simulink model "Plugin_NLPID"  (Simulink 7.3)
settings: Solver=ode45  StartTime=0.0  StopTime=10.0  RelTol=1e-3
libraries: dspmtrx3 x5
settings Model: Creator=mcl  LastModifiedBy=mcl

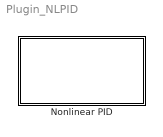
== system Plugin_NLPID ==
  Nonlinear PID : Subsystem

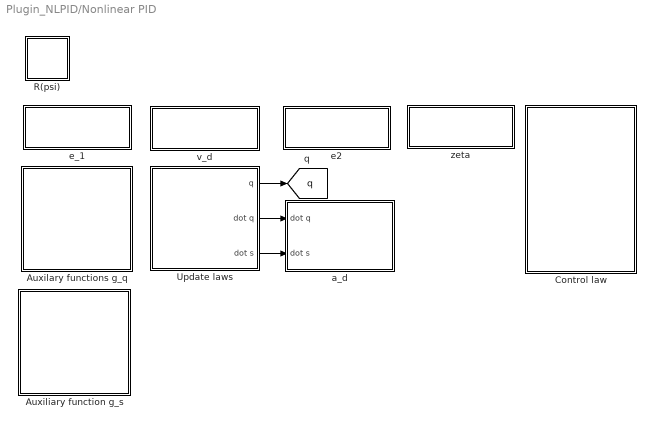
== system Plugin_NLPID/Nonlinear PID ==
  Auxilary functions g_q : Subsystem
  Auxiliary function g_s : Subsystem
  Control law : Subsystem
  R(psi) : Subsystem
  Update laws : Subsystem
  a_d : Subsystem
  e2 : Subsystem
  e_1 : Subsystem
  v_d : Subsystem
  zeta : Subsystem
  tag scope: q=global
  wires:
  Update laws/1(q) -> [q]
  Update laws/2(dot q) -> a_d/1(dot q)
  Update laws/3(dot s) -> a_d/2(dot s)

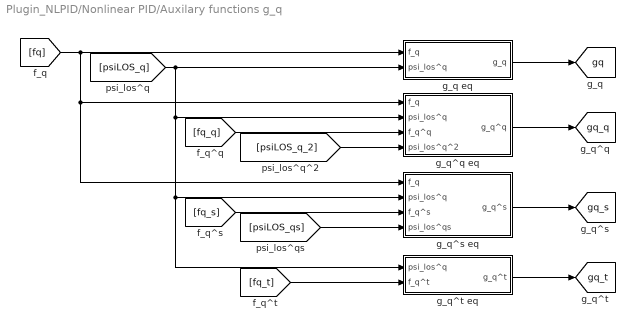
== system Plugin_NLPID/Nonlinear PID/Auxilary functions g_q ==
  g_q eq : Subsystem
  g_q^q eq : Subsystem
  g_q^s eq : Subsystem
  g_q^t eq : Subsystem
  tag scope: gq=global, gq_q=global, gq_s=global, gq_t=global
  wires:
  [fq_t] -> g_q^t eq/2(f_q^t)
  g_q^t eq/1(g_q^t) -> [gq_t]
  [psiLOS_qs] -> g_q^s eq/4(psi_los^qs)
  [fq_s] -> g_q^s eq/3(f_q^s)
  g_q^s eq/1(g_q^s) -> [gq_s]
  g_q^q eq/1(g_q^q) -> [gq_q]
  [psiLOS_q_2] -> g_q^q eq/4(psi_los^q^2)
  [fq_q] -> g_q^q eq/3(f_q^q)
  [fq] -> g_q^s eq/1(f_q), g_q^q eq/1(f_q), g_q eq/1(f_q)
  [psiLOS_q] -> g_q^t eq/1(psi_los^q), g_q^s eq/2(psi_los^q), g_q^q eq/2(psi_los^q), g_q eq/2(psi_los^q)
  g_q eq/1(g_q) -> [gq]

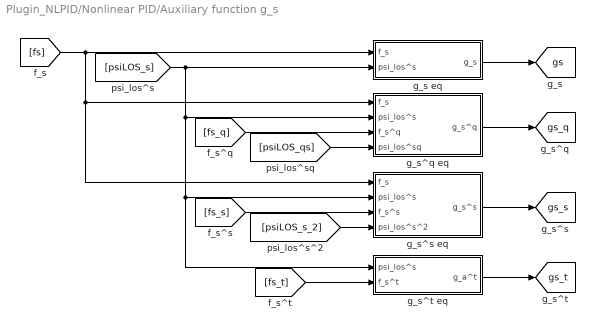
== system Plugin_NLPID/Nonlinear PID/Auxiliary function g_s ==
  g_s eq : Subsystem
  g_s^q eq : Subsystem
  g_s^s eq : Subsystem
  g_s^t eq : Subsystem
  tag scope: gs=global, gs_q=global, gs_s=global, gs_t=global
  wires:
  [fs_t] -> g_s^t eq/2(f_s^t)
  g_s^t eq/1(g_a^t) -> [gs_t]
  [psiLOS_s_2] -> g_s^s eq/4(psi_los^s^2)
  [fs_s] -> g_s^s eq/3(f_s^s)
  g_s^s eq/1(g_s^s) -> [gs_s]
  g_s^q eq/1(g_s^q) -> [gs_q]
  [psiLOS_qs] -> g_s^q eq/4(psi_los^sq)
  [fs_q] -> g_s^q eq/3(f_s^q)
  g_s eq/1(g_s) -> [gs]
  [psiLOS_s] -> g_s^t eq/1(psi_los^s), g_s^s eq/2(psi_los^s), g_s^q eq/2(psi_los^s), g_s eq/2(psi_los^s)
  [fs] -> g_s^s eq/1(f_s), g_s^q eq/1(f_s), g_s eq/1(f_s)

== system Plugin_NLPID/Nonlinear PID/Control law ==
  Product : Product  OutDataType=fixdt(1, 16)  OutScaling=2^0  RndMeth=Zero
  Product1 : Product  OutDataType=fixdt(1, 16)  OutScaling=2^0  RndMeth=Zero
  Sum : Sum  Inputs=+++  OutDataType=fixdt(1, 16)  OutScaling=2^-10
  tau_FF : Subsystem
  tau_FL : Subsystem
  tau_PID : Subsystem
  tag scope: ctrl2tau=global
  wires:
  Sum/1 -> [ctrl2tau]
  tau_PID/1(tau_PID) -> Sum/1
  [tauxscale] -> Product/1
  [tauyscale] -> Product1/1
  tau_FL/1(tau_FL) -> Product/2
  Product/1 -> Sum/2
  tau_FF/1(tau_FF) -> Product1/2
  Product1/1 -> Sum/3

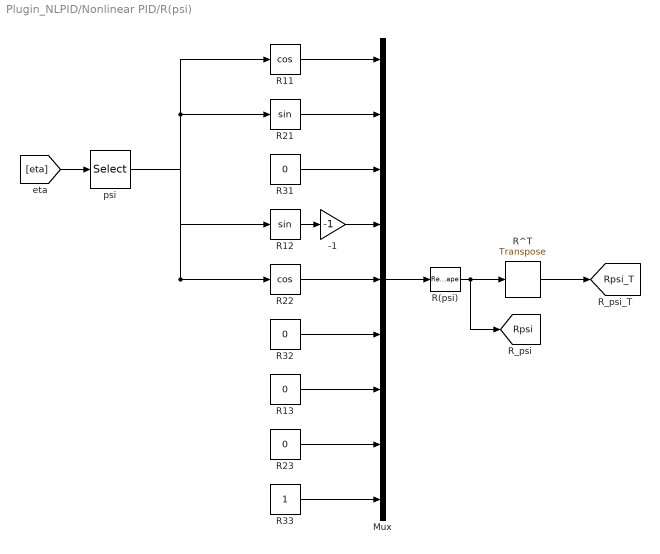
== system Plugin_NLPID/Nonlinear PID/R(psi) ==
  -1 : Gain  Gain=-1  ParameterDataType=fixdt(1, 16)  ParameterScaling=2^0  OutDataType=fixdt(1, 16)  OutScaling=2^0
  Mux : Mux  Inputs=9
  R(psi) : Reshape  OutputDimensionality=Customize  OutputDimensions=[3,3]
  R11 : Trigonometry  Operator=cos
  R12 : Trigonometry
  R{13,23,31..32} (4 alike) : Constant  Value=0
  R21 : Trigonometry
  R22 : Trigonometry  Operator=cos
  R33 : Constant
  R^T : dspmtrx3/Transpose  SystemSampleTime=-1  Hermitian=off  overflowFlag=off
  psi : Selector  InputPortWidth=3  IndexOptions=Index vector (dialog)  Indices=[3]  OutputSizes=1
  tag scope: Rpsi=global, Rpsi_T=global
  wires:
  R(psi)/1 -> [Rpsi], R^T/1
  Mux/1 -> R(psi)/1
  psi/1 -> R11/1, R21/1, R12/1, R22/1
  R11/1 -> Mux/1
  R21/1 -> Mux/2
  R31/1 -> Mux/3
  R12/1 -> -1/1
  R22/1 -> Mux/5
  R32/1 -> Mux/6
  R13/1 -> Mux/7
  R33/1 -> Mux/9
  R23/1 -> Mux/8
  -1/1 -> Mux/4
  [eta] -> psi/1
  R^T/1 -> [Rpsi_T]

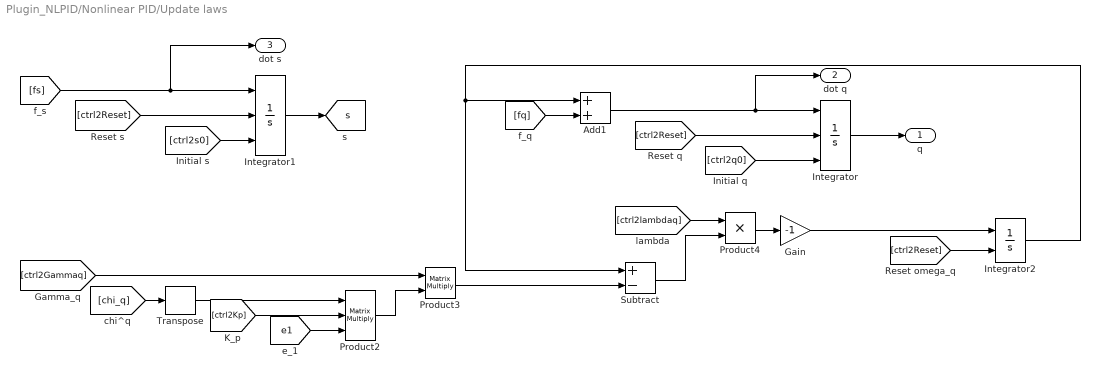
== system Plugin_NLPID/Nonlinear PID/Update laws ==
  Add1 : Sum  OutDataType=fixdt(1, 16)  OutScaling=2^-10
  Gain : Gain  Gain=-1  ParameterDataType=fixdt(1, 16)  ParameterScaling=2^0  OutDataType=fixdt(1, 16)  OutScaling=2^0
  Integrator : Integrator  ExternalReset=level  InitialConditionSource=external
  Integrator1 : Integrator  ExternalReset=level  InitialConditionSource=external  InitialCondition=250
  Integrator2 : Integrator  ExternalReset=level
  Product2 : Product  Inputs=3  Multiplication=Matrix(*)  OutDataType=fixdt(1, 16)  OutScaling=2^0  RndMeth=Zero
  Product3 : Product  Multiplication=Matrix(*)  OutDataType=fixdt(1, 16)  OutScaling=2^0  RndMeth=Zero
  Product4 : Product  OutDataType=fixdt(1, 16)  OutScaling=2^0  RndMeth=Zero
  Subtract : Sum  Inputs=+-  OutDataType=fixdt(1, 16)  OutScaling=2^-10
  Transpose : dspmtrx3/Transpose  SystemSampleTime=-1  Hermitian=off  overflowFlag=off
  q : Outport  PortDimensions=2
  dot q : Outport  Port=2  PortDimensions=2
  dot s : Outport  Port=3  PortDimensions=1
  tag scope: s=global
  wires:
  [chi_q] -> Transpose/1
  [e1] -> Product2/3
  Transpose/1 -> Product2/1
  [ctrl2Kp] -> Product2/2
  [ctrl2Gammaq] -> Product3/1
  Product3/1 -> Subtract/2
  Product2/1 -> Product3/2
  [fs] -> Integrator1/1, dot s/1
  Integrator1/1 -> [s]
  [ctrl2Reset] -> Integrator1/2
  [ctrl2s0] -> Integrator1/3
  [fq] -> Add1/2
  Add1/1 -> Integrator/1, dot q/1
  [ctrl2lambdaq] -> Product4/1
  Subtract/1 -> Product4/2
  Product4/1 -> Gain/1
  Gain/1 -> Integrator2/1
  Integrator/1 -> q/1
  Integrator2/1 -> Add1/1, Subtract/1
  [ctrl2Reset] -> Integrator/2
  [ctrl2q0] -> Integrator/3
  [ctrl2Reset] -> Integrator2/2

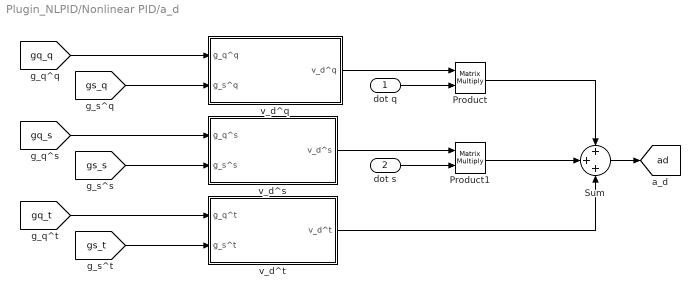
== system Plugin_NLPID/Nonlinear PID/a_d ==
  dot q : Inport
  dot s : Inport  Port=2
  Product : Product  Multiplication=Matrix(*)  OutDataType=fixdt(1, 16)  OutScaling=2^0  RndMeth=Zero
  Product1 : Product  Multiplication=Matrix(*)  OutDataType=fixdt(1, 16)  OutScaling=2^0  RndMeth=Zero
  Sum : Sum  Inputs=+++  OutDataType=fixdt(1, 16)  OutScaling=2^-10
  v_d^q : Subsystem
  v_d^s : Subsystem
  v_d^t : Subsystem
  tag scope: ad=global
  wires:
  v_d^q/1(v_d^q) -> Product/1
  dot q/1 -> Product/2
  Product/1 -> Sum/1
  v_d^s/1(v_d^s) -> Product1/1
  dot s/1 -> Product1/2
  Product1/1 -> Sum/2
  v_d^t/1(v_d^t) -> Sum/3
  Sum/1 -> [ad]
  [gq_q] -> v_d^q/1(g_q^q)
  [gs_q] -> v_d^q/2(g_s^q)
  [gq_s] -> v_d^s/1(g_q^s)
  [gs_s] -> v_d^s/2(g_s^s)
  [gq_t] -> v_d^t/1(g_q^t)
  [gs_t] -> v_d^t/2(g_s^t)

== system Plugin_NLPID/Nonlinear PID/e2 ==
  Product : Product  Multiplication=Matrix(*)  OutDataType=fixdt(1, 16)  OutScaling=2^0  RndMeth=Zero
  Subtract : Sum  Inputs=+-  OutDataType=fixdt(1, 16)  OutScaling=2^-10
  tag scope: e2=global
  wires:
  [nu] -> Subtract/1
  Product/1 -> Subtract/2
  [Rpsi_T] -> Product/1
  [vd] -> Product/2
  Subtract/1 -> [e2]

== system Plugin_NLPID/Nonlinear PID/e_1 ==
  Heading to -pi/pi : Subsystem
  Heading to -pi/pi1 : Subsystem
  Subtract : Sum  Inputs=+-  OutDataType=fixdt(1, 16)  OutScaling=2^-10
  tag scope: e1=global
  wires:
  Subtract/1 -> Heading to -pi/pi1/1(eta rad)
  [eta] -> Heading to -pi/pi/1(eta rad)
  Heading to -pi/pi/1(eta -pi/pi) -> Subtract/1
  Heading to -pi/pi1/1(eta -pi/pi) -> [e1]
  [chi] -> Subtract/2

== system Plugin_NLPID/Nonlinear PID/v_d ==
  Add : Sum  OutDataType=fixdt(1, 16)  OutScaling=2^-10
  tag scope: vd=global
  wires:
  [gq] -> Add/1
  [gs] -> Add/2
  Add/1 -> [vd]

== system Plugin_NLPID/Nonlinear PID/zeta ==
  Integrator : Integrator  ExternalReset=level  InitialCondition=[0 0 0]'
  Product : Product  Multiplication=Matrix(*)  OutDataType=fixdt(1, 16)  OutScaling=2^0  RndMeth=Zero
  tag scope: zeta=global
  wires:
  [ctrl2Reset] -> Integrator/2
  Product/1 -> Integrator/1
  Integrator/1 -> [zeta]
  [e2] -> Product/2
  [Rpsi] -> Product/1

== system Plugin_NLPID/Nonlinear PID/Auxilary functions g_q/g_q eq ==
  f_q : Inport
  psi_los^q : Inport  Port=2
  Product : Product  Multiplication=Matrix(*)  OutDataType=fixdt(1, 16)  OutScaling=2^0  RndMeth=Zero
  Vector Concatenate : Concatenate  Mode=Vector
  g_q : Outport
  wires:
  Product/1 -> Vector Concatenate/2
  psi_los^q/1 -> Product/1
  f_q/1 -> Product/2, Vector Concatenate/1
  Vector Concatenate/1 -> g_q/1

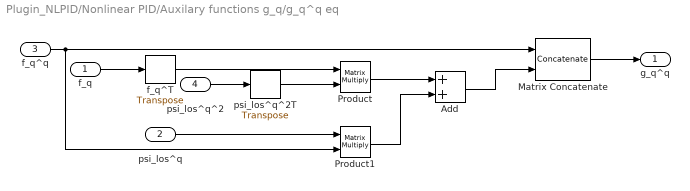
== system Plugin_NLPID/Nonlinear PID/Auxilary functions g_q/g_q^q eq ==
  f_q : Inport
  psi_los^q : Inport  Port=2
  f_q^q : Inport  Port=3
  psi_los^q^2 : Inport  Port=4
  Add : Sum  OutDataType=fixdt(1, 16)  OutScaling=2^-10
  Matrix Concatenate : Concatenate  Mode=Multidimensional array
  Product : Product  Multiplication=Matrix(*)  OutDataType=fixdt(1, 16)  OutScaling=2^0  RndMeth=Zero
  Product1 : Product  Multiplication=Matrix(*)  OutDataType=fixdt(1, 16)  OutScaling=2^0  RndMeth=Zero
  f_q^T : dspmtrx3/Transpose  SystemSampleTime=-1  Hermitian=off  overflowFlag=off
  psi_los^q^2T : dspmtrx3/Transpose  SystemSampleTime=-1  Hermitian=off  overflowFlag=off
  g_q^q : Outport
  wires:
  psi_los^q^2T/1 -> Product/2
  Product1/1 -> Add/2
  psi_los^q/1 -> Product1/1
  Product/1 -> Add/1
  psi_los^q^2/1 -> psi_los^q^2T/1
  f_q^T/1 -> Product/1
  f_q/1 -> f_q^T/1
  Add/1 -> Matrix Concatenate/2
  Matrix Concatenate/1 -> g_q^q/1
  f_q^q/1 -> Product1/2, Matrix Concatenate/1

== system Plugin_NLPID/Nonlinear PID/Auxilary functions g_q/g_q^s eq ==
  f_q : Inport
  psi_los^q : Inport  Port=2
  f_q^s : Inport  Port=3
  psi_los^qs : Inport  Port=4
  Add : Sum  OutDataType=fixdt(1, 16)  OutScaling=2^-10
  Product : Product  Multiplication=Matrix(*)  OutDataType=fixdt(1, 16)  OutScaling=2^0  RndMeth=Zero
  Product1 : Product  Multiplication=Matrix(*)  OutDataType=fixdt(1, 16)  OutScaling=2^0  RndMeth=Zero
  Vector Concatenate : Concatenate  Mode=Vector
  g_q^s : Outport
  wires:
  f_q/1 -> Product/2
  psi_los^qs/1 -> Product/1
  Product1/1 -> Add/2
  psi_los^q/1 -> Product1/1
  Product/1 -> Add/1
  Add/1 -> Vector Concatenate/2
  Vector Concatenate/1 -> g_q^s/1
  f_q^s/1 -> Product1/2, Vector Concatenate/1

== system Plugin_NLPID/Nonlinear PID/Auxilary functions g_q/g_q^t eq ==
  psi_los^q : Inport
  f_q^t : Inport  Port=2
  Product1 : Product  Multiplication=Matrix(*)  OutDataType=fixdt(1, 16)  OutScaling=2^0  RndMeth=Zero
  Vector Concatenate : Concatenate  Mode=Vector
  g_q^t : Outport
  wires:
  psi_los^q/1 -> Product1/1
  Product1/1 -> Vector Concatenate/2
  Vector Concatenate/1 -> g_q^t/1
  f_q^t/1 -> Product1/2, Vector Concatenate/1

== system Plugin_NLPID/Nonlinear PID/Auxiliary function g_s/g_s eq ==
  f_s : Inport
  psi_los^s : Inport  Port=2
  0_2x1 : Constant  Value=[0;0]  VectorParams1D=off  OutDataType=fixdt(1, 16)  OutScaling=2^0
  Product : Product  Multiplication=Matrix(*)  OutDataType=fixdt(1, 16)  OutScaling=2^0  RndMeth=Zero
  Vector Concatenate : Concatenate  Mode=Vector
  g_s : Outport
  wires:
  0_2x1/1 -> Vector Concatenate/1
  Product/1 -> Vector Concatenate/2
  psi_los^s/1 -> Product/1
  f_s/1 -> Product/2
  Vector Concatenate/1 -> g_s/1

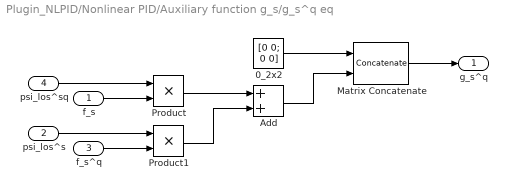
== system Plugin_NLPID/Nonlinear PID/Auxiliary function g_s/g_s^q eq ==
  f_s : Inport
  psi_los^s : Inport  Port=2
  f_s^q : Inport  Port=3
  psi_los^sq : Inport  Port=4
  0_2x2 : Constant  Value=[0 0; 0 0]  VectorParams1D=off  OutDataType=fixdt(1, 16)  OutScaling=2^0
  Add : Sum  OutDataType=fixdt(1, 16)  OutScaling=2^-10
  Matrix Concatenate : Concatenate  Mode=Multidimensional array
  Product : Product  OutDataType=fixdt(1, 16)  OutScaling=2^0  RndMeth=Zero
  Product1 : Product  OutDataType=fixdt(1, 16)  OutScaling=2^0  RndMeth=Zero
  g_s^q : Outport
  wires:
  f_s/1 -> Product/2
  psi_los^sq/1 -> Product/1
  f_s^q/1 -> Product1/2
  0_2x2/1 -> Matrix Concatenate/1
  Product1/1 -> Add/2
  psi_los^s/1 -> Product1/1
  Product/1 -> Add/1
  Add/1 -> Matrix Concatenate/2
  Matrix Concatenate/1 -> g_s^q/1

== system Plugin_NLPID/Nonlinear PID/Auxiliary function g_s/g_s^s eq ==
  f_s : Inport
  psi_los^s : Inport  Port=2
  f_s^s : Inport  Port=3
  psi_los^s^2 : Inport  Port=4
  0_2x1 : Constant  Value=[0;0]  VectorParams1D=off  OutDataType=fixdt(1, 16)  OutScaling=2^0
  Add : Sum  OutDataType=fixdt(1, 16)  OutScaling=2^-10
  Product : Product  OutDataType=fixdt(1, 16)  OutScaling=2^0  RndMeth=Zero
  Product1 : Product  OutDataType=fixdt(1, 16)  OutScaling=2^0  RndMeth=Zero
  Vector Concatenate : Concatenate  Mode=Vector
  g_s^s : Outport
  wires:
  f_s^s/1 -> Product1/2
  0_2x1/1 -> Vector Concatenate/1
  f_s/1 -> Product/2
  psi_los^s^2/1 -> Product/1
  Product1/1 -> Add/2
  psi_los^s/1 -> Product1/1
  Product/1 -> Add/1
  Add/1 -> Vector Concatenate/2
  Vector Concatenate/1 -> g_s^s/1

== system Plugin_NLPID/Nonlinear PID/Auxiliary function g_s/g_s^t eq ==
  psi_los^s : Inport
  f_s^t : Inport  Port=2
  0_2x1 : Constant  Value=[0;0]  VectorParams1D=off  OutDataType=fixdt(1, 16)  OutScaling=2^0
  Product1 : Product  Multiplication=Matrix(*)  OutDataType=fixdt(1, 16)  OutScaling=2^0  RndMeth=Zero
  Vector Concatenate : Concatenate  Mode=Vector
  g_a^t : Outport
  wires:
  f_s^t/1 -> Product1/2
  0_2x1/1 -> Vector Concatenate/1
  psi_los^s/1 -> Product1/1
  Product1/1 -> Vector Concatenate/2
  Vector Concatenate/1 -> g_a^t/1

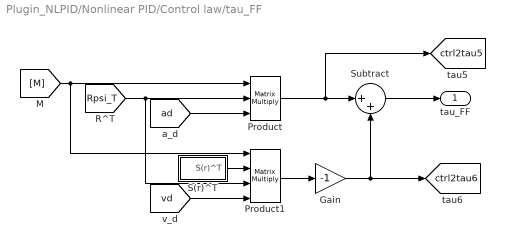
== system Plugin_NLPID/Nonlinear PID/Control law/tau_FF ==
  Gain : Gain  Gain=-1  ParameterDataType=fixdt(1, 16)  ParameterScaling=2^0  OutDataType=fixdt(1, 16)  OutScaling=2^0
  Product : Product  Inputs=3  Multiplication=Matrix(*)  OutDataType=fixdt(1, 16)  OutScaling=2^0  RndMeth=Zero
  Product1 : Product  Inputs=4  Multiplication=Matrix(*)  OutDataType=fixdt(1, 16)  OutScaling=2^0  RndMeth=Zero
  S(r)^T : Subsystem
  Subtract : Sum  Inputs=|++  OutDataType=fixdt(1, 16)  OutScaling=2^-10
  tau_FF : Outport
  tag scope: ctrl2tau5=global, ctrl2tau6=global
  wires:
  Subtract/1 -> tau_FF/1
  [Rpsi_T] -> Product/2, Product1/3
  [ad] -> Product/3
  Product/1 -> Subtract/1, [ctrl2tau5]
  Product1/1 -> Gain/1
  S(r)^T/1(S(r)^T) -> Product1/2
  [vd] -> Product1/4
  [M] -> Product/1, Product1/1
  Gain/1 -> Subtract/2, [ctrl2tau6]

== system Plugin_NLPID/Nonlinear PID/Control law/tau_FL ==
  Product1 : Product  Multiplication=Matrix(*)  OutDataType=fixdt(1, 16)  OutScaling=2^0  RndMeth=Zero
  tau_FL : Outport
  tag scope: ctrl2tau4=global
  wires:
  [DL] -> Product1/1
  Product1/1 -> tau_FL/1, [ctrl2tau4]
  [nu] -> Product1/2

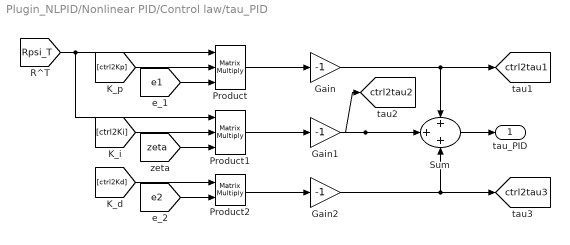
== system Plugin_NLPID/Nonlinear PID/Control law/tau_PID ==
  Gain : Gain  Gain=-1  ParameterDataType=fixdt(1, 16)  ParameterScaling=2^0  OutDataType=fixdt(1, 16)  OutScaling=2^0
  Gain1 : Gain  Gain=-1  ParameterDataType=fixdt(1, 16)  ParameterScaling=2^0  OutDataType=fixdt(1, 16)  OutScaling=2^0
  Gain2 : Gain  Gain=-1  ParameterDataType=fixdt(1, 16)  ParameterScaling=2^0  OutDataType=fixdt(1, 16)  OutScaling=2^0
  Product : Product  Inputs=3  Multiplication=Matrix(*)  OutDataType=fixdt(1, 16)  OutScaling=2^0  RndMeth=Zero
  Product1 : Product  Inputs=3  Multiplication=Matrix(*)  OutDataType=fixdt(1, 16)  OutScaling=2^0  RndMeth=Zero
  Product2 : Product  Multiplication=Matrix(*)  OutDataType=fixdt(1, 16)  OutScaling=2^0  RndMeth=Zero
  Sum : Sum  Inputs=+++  OutDataType=fixdt(1, 16)  OutScaling=2^-10
  tau_PID : Outport
  tag scope: ctrl2tau1=global, ctrl2tau2=global, ctrl2tau3=global
  wires:
  [Rpsi_T] -> Product/1, Product1/1
  [ctrl2Kp] -> Product/2
  [e1] -> Product/3
  [ctrl2Ki] -> Product1/2
  [zeta] -> Product1/3
  [ctrl2Kd] -> Product2/1
  [e2] -> Product2/2
  Sum/1 -> tau_PID/1
  Product/1 -> Gain/1
  Product1/1 -> Gain1/1
  Product2/1 -> Gain2/1
  Gain/1 -> Sum/1, [ctrl2tau1]
  Gain1/1 -> Sum/2, [ctrl2tau2]
  Gain2/1 -> Sum/3, [ctrl2tau3]

== system Plugin_NLPID/Nonlinear PID/a_d/v_d^q ==
  g_q^q : Inport
  g_s^q : Inport  Port=2
  Add : Sum  OutDataType=fixdt(1, 16)  OutScaling=2^-10
  v_d^q : Outport
  wires:
  Add/1 -> v_d^q/1
  g_q^q/1 -> Add/1
  g_s^q/1 -> Add/2

== system Plugin_NLPID/Nonlinear PID/a_d/v_d^s ==
  g_q^s : Inport
  g_s^s : Inport  Port=2
  Add1 : Sum  OutDataType=fixdt(1, 16)  OutScaling=2^-10
  v_d^s : Outport
  wires:
  Add1/1 -> v_d^s/1
  g_q^s/1 -> Add1/1
  g_s^s/1 -> Add1/2

== system Plugin_NLPID/Nonlinear PID/a_d/v_d^t ==
  g_q^t : Inport
  g_s^t : Inport  Port=2
  Add : Sum  OutDataType=fixdt(1, 16)  OutScaling=2^-10
  v_d^t : Outport
  wires:
  Add/1 -> v_d^t/1
  g_q^t/1 -> Add/1
  g_s^t/1 -> Add/2

== system Plugin_NLPID/Nonlinear PID/e_1/Heading to -pi/pi ==
  eta rad : Inport
  Demux : Demux  Outputs=3
  Mux : Mux  Inputs=3
  rad to [-pi pi] : Subsystem
      mask Type: rad to pi/pi
      mask Description: Converts an angle in rad to between -pi and pi
      mask Display: disp('rad to [-pi pi]')
  eta -pi/pi : Outport
  wires:
  rad to [-pi pi]/1("[-pi pi]") -> Mux/3
  Mux/1 -> eta -pi/pi/1
  eta rad/1 -> Demux/1
  Demux/2 -> Mux/2
  Demux/1 -> Mux/1
  Demux/3 -> rad to [-pi pi]/1(rad)

== system Plugin_NLPID/Nonlinear PID/e_1/Heading to -pi/pi1 ==
  eta rad : Inport
  Demux : Demux  Outputs=3
  Mux : Mux  Inputs=3
  rad to [-pi pi] : Subsystem
      mask Type: rad to pi/pi
      mask Description: Converts an angle in rad to between -pi and pi
      mask Display: disp('rad to [-pi pi]')
  eta -pi/pi : Outport
  wires:
  rad to [-pi pi]/1("[-pi pi]") -> Mux/3
  Mux/1 -> eta -pi/pi/1
  eta rad/1 -> Demux/1
  Demux/2 -> Mux/2
  Demux/1 -> Mux/1
  Demux/3 -> rad to [-pi pi]/1(rad)

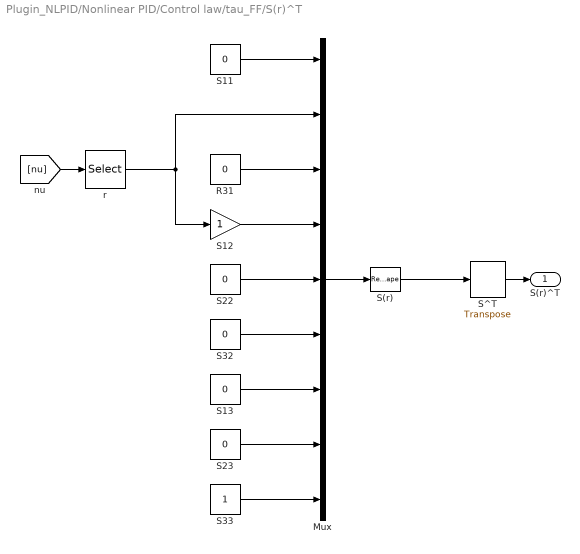
== system Plugin_NLPID/Nonlinear PID/Control law/tau_FF/S(r)^T ==
  Mux : Mux  Inputs=9
  R31 : Constant  Value=0
  S(r) : Reshape  OutputDimensionality=Customize  OutputDimensions=[3,3]
  S{11,13,22..23,32} (5 alike) : Constant  Value=0
  S12 : Gain  ParameterDataType=fixdt(1, 16)  ParameterScaling=2^0  OutDataType=fixdt(1, 16)  OutScaling=2^0
  S33 : Constant
  S^T : dspmtrx3/Transpose  SystemSampleTime=-1  Hermitian=off  overflowFlag=off
  r : Selector  InputPortWidth=3  IndexOptions=Index vector (dialog)  Indices=[3]  OutputSizes=1
  S(r)^T : Outport
  wires:
  S(r)/1 -> S^T/1
  Mux/1 -> S(r)/1
  R31/1 -> Mux/3
  S12/1 -> Mux/4
  S22/1 -> Mux/5
  S32/1 -> Mux/6
  S13/1 -> Mux/7
  S33/1 -> Mux/9
  S23/1 -> Mux/8
  S11/1 -> Mux/1
  r/1 -> Mux/2, S12/1
  [nu] -> r/1
  S^T/1 -> S(r)^T/1

== system Plugin_NLPID/Nonlinear PID/e_1/Heading to -pi/pi/rad to [-pi pi] ==
  rad : Inport  OutDataType=sfix(16)  OutScaling=2^0
  Constant : Constant  Value=2*pi  OutDataType=sfix(16)  OutScaling=2^0
  Gain : Gain  Gain=pi  ParameterDataType=sfix(16)  ParameterScaling=2^0  OutDataType=sfix(16)  OutScaling=2^0  SaturateOnIntegerOverflow=on  OutDataTypeStr=Inherit: Same as input  ParamDataTypeStr=Inherit: Same as input
  Math Function : Math  Operator=rem  OutDataType=sfix(16)  OutScaling=2^0  SaturateOnIntegerOverflow=on
  Saturation : Saturate  UpperLimit=1e10  LowerLimit=-1e10
  Sign : Signum
  Sum : Sum  Inputs=|+-  OutDataType=sfix(16)  OutScaling=2^0  SaturateOnIntegerOverflow=on
  Sum1 : Sum  Inputs=|++  OutDataType=sfix(16)  OutScaling=2^0  SaturateOnIntegerOverflow=on
  "[-pi pi]" : Outport  OutDataType=sfix(16)  OutScaling=2^0
  wires:
  Sum/1 -> "[-pi pi]"/1
  Math Function/1 -> Sum/1
  Constant/1 -> Math Function/2
  Sum1/1 -> Math Function/1
  Gain/1 -> Sum1/2, Sum/2
  Sign/1 -> Gain/1
  rad/1 -> Saturation/1
  Saturation/1 -> Sign/1, Sum1/1

== system Plugin_NLPID/Nonlinear PID/e_1/Heading to -pi/pi1/rad to [-pi pi] ==
  rad : Inport  OutDataType=sfix(16)  OutScaling=2^0
  Constant : Constant  Value=2*pi  OutDataType=sfix(16)  OutScaling=2^0
  Gain : Gain  Gain=pi  ParameterDataType=sfix(16)  ParameterScaling=2^0  OutDataType=sfix(16)  OutScaling=2^0  SaturateOnIntegerOverflow=on  OutDataTypeStr=Inherit: Same as input  ParamDataTypeStr=Inherit: Same as input
  Math Function : Math  Operator=rem  OutDataType=sfix(16)  OutScaling=2^0  SaturateOnIntegerOverflow=on
  Saturation : Saturate  UpperLimit=1e10  LowerLimit=-1e10
  Sign : Signum
  Sum : Sum  Inputs=|+-  OutDataType=sfix(16)  OutScaling=2^0  SaturateOnIntegerOverflow=on
  Sum1 : Sum  Inputs=|++  OutDataType=sfix(16)  OutScaling=2^0  SaturateOnIntegerOverflow=on
  "[-pi pi]" : Outport  OutDataType=sfix(16)  OutScaling=2^0
  wires:
  Sum/1 -> "[-pi pi]"/1
  Math Function/1 -> Sum/1
  Constant/1 -> Math Function/2
  Sum1/1 -> Math Function/1
  Gain/1 -> Sum1/2, Sum/2
  Sign/1 -> Gain/1
  rad/1 -> Saturation/1
  Saturation/1 -> Sign/1, Sum1/1
